simulink model "DiagramaDCarmadura"  (R2017b)
settings: Solver=VariableStepAuto  StartTime=0.0  StopTime=10.0  RelTol=1e-3
values from neighbouring files (symbols this model uses):
  B = 0.002953    [Graficas.m]
  J = 0.0221    [Graficas.m]
  Kb = 1.25    [Graficas.m]
  Kt = 0.516    [Graficas.m]
  La = 0.0281    [Graficas.m]
  Ra = 2.581    [Graficas.m]
  ST = 1    [Graficas.m]
  Td = 0    [Graficas.m]
  VF = 240    [Graficas.m]
  VI = 140    [Graficas.m]
settings Model: Creator=usuario  LastModifiedBy=Wilmer
settings SFSimCC: SimUseLocalCustomCode=on
settings RTWCC: RTWUseLocalCustomCode=on
settings CodeAppCC: StateflowObjectComments=on

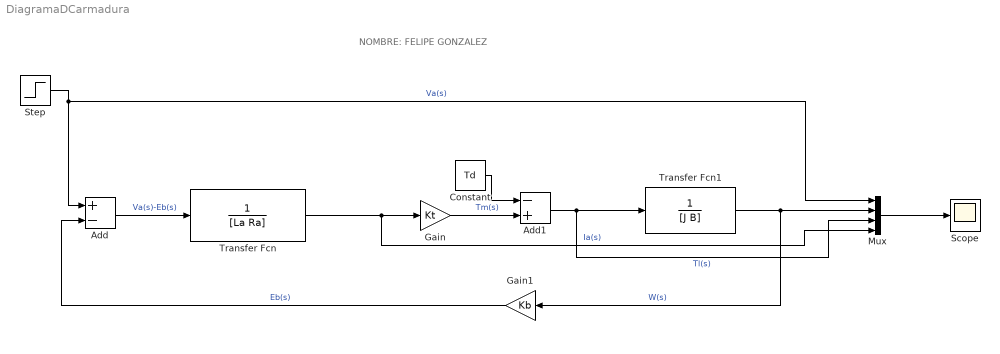
== system DiagramaDCarmadura ==
  note: NOMBRE: FELIPE GONZALEZ
  Add : Sum  Inputs=+-
  Add1 : Sum  Inputs=-+
  Constant : Constant  Value=Td
  Gain : Gain  Gain=Kt
  Gain1 : Gain  Gain=Kb
  Mux : Mux
  Scope : Scope
  Step : Step  Time=ST  Before=VI  After=VF  SampleTime=0
  Transfer Fcn : TransferFcn  Denominator=[La Ra]
  Transfer Fcn1 : TransferFcn  Denominator=[J B]
  wires:
  Step/1 -> Mux/1, Add/1  "Va(s)"
  Gain1/1 -> Add/2  "Eb(s)"
  Add/1 -> Transfer Fcn/1  "Va(s)-Eb(s)"
  Transfer Fcn/1 -> Mux/4, Gain/1  "Ia(s)"
  Gain/1 -> Add1/2  "Tm(s)"
  Constant/1 -> Add1/1
  Add1/1 -> Mux/3, Transfer Fcn1/1  "Tl(s)"
  Transfer Fcn1/1 -> Mux/2, Gain1/1  "W(s)"
  Mux/1 -> Scope/1
